simulink model "Pendulum_Motion_2021b"  (R2021b)
settings: Solver=VariableStepAuto  StartTime=0.0  StopTime=10.0  MaxStep=1e-3  RelTol=1e-3
values from neighbouring files (symbols this model uses):
  g = 9.8    [Pendulum__Motion.m]
  Initial_displacement = 0    [Pendulum__Motion.m]
  Initial_Velocity = 0.1    [Pendulum__Motion.m]
  L = Length(i)    [Pendulum__Motion.m]
settings Model: Creator=gaafa  LastModifiedBy=gaafa
settings DebuggingCC: UnconnectedInputMsg=none  UnconnectedOutputMsg=none  UnconnectedLineMsg=none
settings ModelReferenceCC: EnableRefExpFcnMdlSchedulingChecks=off
settings RTWCC: DLArmComputeVersion=20.02.1

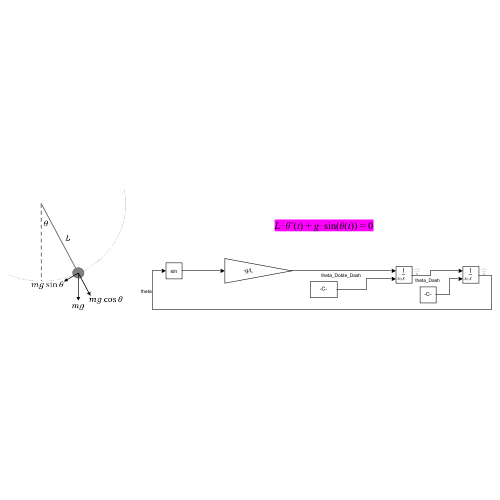
[thumbnail: Simulink's stored preview of the top-level diagram]
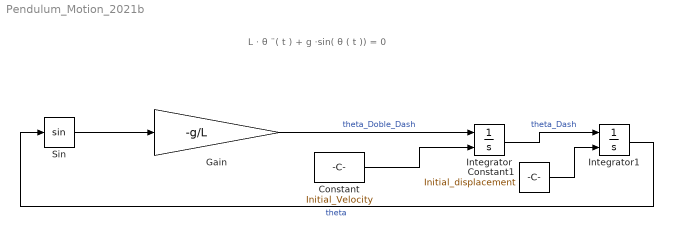
== system Pendulum_Motion_2021b ==
  note: L ⋅ θ ¨( t ) + g ⋅sin( θ ( t )) = 0
  Constant : Constant  Value=Initial_Velocity
  Constant1 : Constant  Value=Initial_displacement
  Gain : Gain  Gain=-g/L
  Integrator : Integrator  InitialConditionSource=external  InitialCondition=0.1
  Integrator1 : Integrator  InitialConditionSource=external
  Sin : Trigonometry
  wires:
  Integrator1/1 -> Sin/1  "theta"
  Sin/1 -> Gain/1
  Gain/1 -> Integrator/1  "theta_Doble_Dash"
  Integrator/1 -> Integrator1/1  "theta_Dash"
  Constant/1 -> Integrator/2
  Constant1/1 -> Integrator1/2
